simulink model "quad_lqr_only"  (R2023b)
settings: Solver=VariableStepAuto  StartTime=0.0  StopTime=100  RelTol=1e-3
values from neighbouring files (symbols this model uses):
  K2 = lqr(sys,Q,R)    [model_data.m]
  sys = ss(quad_state_A,quad_actuator_B,observer_C,D)    [lqr_quad_for_body_rate_control_model.m]    (also in lqr_quad_for_euler_rate_control_model.m; model_data.m)
settings Model: NumberOfSteps=10  Creator=karukkuvel-raj  LastModifiedBy=karukkuvel-raj
settings DebuggingCC: AlgebraicLoopMsg=none

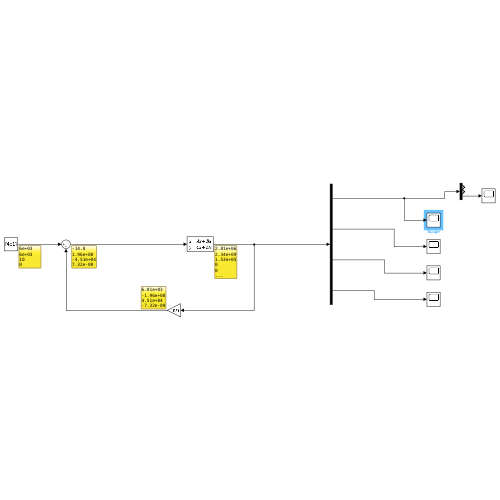
[thumbnail: Simulink's stored preview of the top-level diagram]
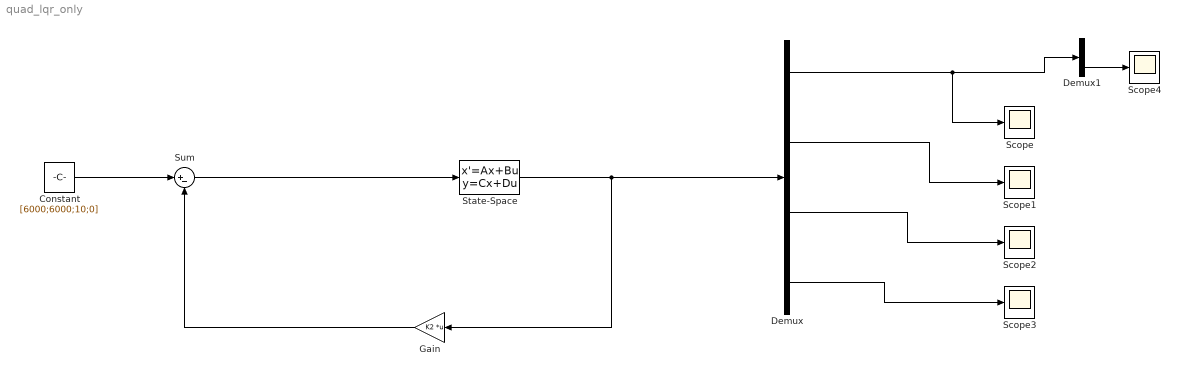
== system quad_lqr_only ==
  Constant : Constant  Value=[6000;6000;10;0]
  Demux : Demux
  Demux1 : Demux  Outputs=3
  Gain : Gain  Gain=K2  Multiplication=Matrix(K*u)
  Scope{,1..4} (5 alike) : Scope
  State-Space : StateSpace  A=sys.A  B=sys.B  C=sys.C  D=sys.D  InitialCondition=0  AllowTunableDMatrix=on
  Sum : Sum  Inputs=|+-
  wires:
  State-Space/1 -> Gain/1, Demux/1
  Demux/1 -> Demux1/1, Scope/1
  Demux/2 -> Scope1/1
  Demux/3 -> Scope2/1
  Demux/4 -> Scope3/1
  Gain/1 -> Sum/2
  Constant/1 -> Sum/1
  Sum/1 -> State-Space/1
  Demux1/3 -> Scope4/1
